simulink model "itki"  (R2019b)
settings: Solver=VariableStepAuto  StartTime=0.0  StopTime=1000  RelTol=1e-3
model workspace (MAT data in the model file):
  itki = [0 1000 1800 2300 2400 2350 2400 2600 2300 2250 2200 750 150 100 20]
undefined symbols (not defined in the file): Earth, magnitude, WGS84
libraries: dspsrcs4 x3, aerolibfltsims x2, simulink x1, sharedtransform x1, aerolibtransform2 x1
settings Model: Creator=LENOVO  LastModifiedBy=LENOVO

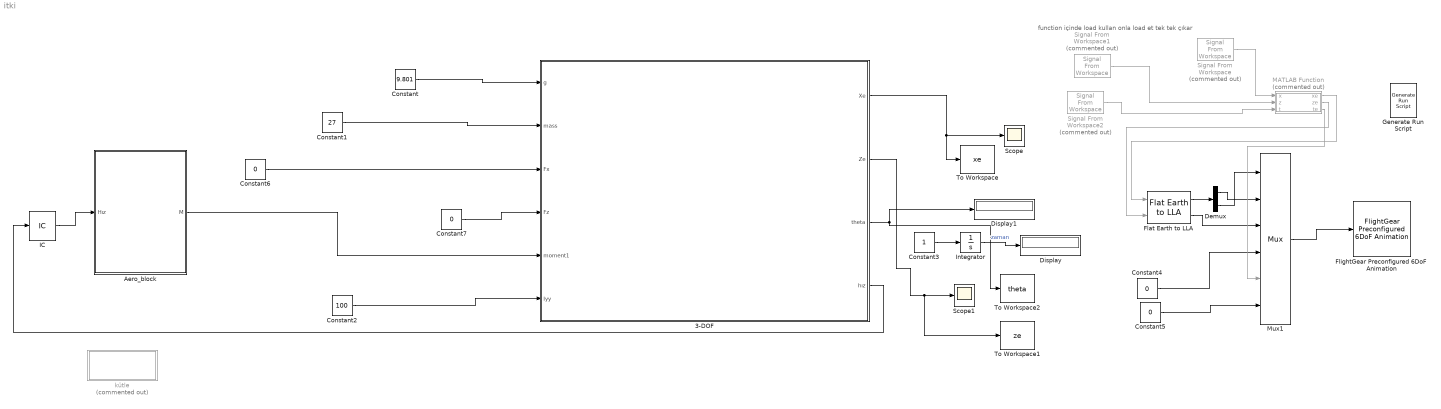
== system itki ==
  note: function içinde load kullan onla load et tek tek çıkar
  3-DOF : Subsystem
  Aero_block : Subsystem
  Constant : Constant  Value=9.801
  Constant1 : Constant  Value=27
  Constant2 : Constant  Value=100
  Constant3 : Constant
  Constant{4..7} (4 alike) : Constant  Value=0
  Demux : Demux  Outputs=2
  Display : Display
  Display1 : Display
  Flat Earth to LLA : aerolibtransform2/Flat Earth to LLA  units=Metric (MKS)  ptype=Earth (WGS84)  F=1/298.257223563  R=6378137  LL0=[0 10]  psi=0
  FlightGear Preconfigured 6DoF Animation : aerolibfltsims/FlightGear Preconfigured 6DoF Animation  xFlightGearVersion=v2018.3  DestinationIpAddress=127.0.0.1  DestinationPort=5502  SampleTime=1/30  packetVersion=24
      settings: SourceProductName=Aerospace Blockset
  Generate Run Script : aerolibfltsims/Generate Run Script  Architecture=Win64  dataFlow=Send  GeometryModelName=HL20  AirportId=KSFO  RunwayId=10L  InitialAltitude=7224  InitialHeading=113  OffsetDistance=4.72  OffsetAzimuth=0  InstallScenery=off  DisableShaders=on  OriginAddress=127.0.0.1  DestinationPort=5502  OriginPort=5505  LocalAddress=127.0.0.1  OutputFileName=runfg.bat  FlightGearBaseDirectory=C:\Program Files\FlightGear 2020.3
  IC : InitialCondition  Value=100
  Integrator : Integrator
  MATLAB Function : MATLAB Function  Commented=on  TreatAsAtomicUnit=on
  Mux1 : Mux  Inputs=6
  Scope : Scope
  Scope1 : Scope
  Signal From Workspace : dspsrcs4/Signal From Workspace  Commented=on  X=out.xe  Ts=0.1  nsamps=1  OutputAfterFinalValue=Setting to zero  ignoreOrWarnInputAndFrameLengths=off  OutputFrames=off
  Signal From Workspace1 : dspsrcs4/Signal From Workspace  Commented=on  X=out.ze  Ts=0.1  nsamps=1  OutputAfterFinalValue=Setting to zero  ignoreOrWarnInputAndFrameLengths=off  OutputFrames=off
  Signal From Workspace2 : dspsrcs4/Signal From Workspace  Commented=on  X=out.theta  Ts=0.1  nsamps=1  OutputAfterFinalValue=Setting to zero  ignoreOrWarnInputAndFrameLengths=off  OutputFrames=off
  To Workspace : ToWorkspace  VariableName=xe  SampleTime=0.1
      settings: Save2DSignal=2-D array (concatenate along first dimension)
  To Workspace1 : ToWorkspace  VariableName=ze  SampleTime=0.1
      settings: Save2DSignal=2-D array (concatenate along first dimension)
  To Workspace2 : ToWorkspace  VariableName=theta  SampleTime=0.1
      settings: Save2DSignal=2-D array (concatenate along first dimension)
  kütle : Subsystem  Commented=on
  wires:
  Constant/1 -> 3-DOF/1(g)
  Constant1/1 -> 3-DOF/2(mass)
  Constant6/1 -> 3-DOF/3(Fx)
  Aero_block/1(M) -> 3-DOF/5(moment1)
  Constant2/1 -> 3-DOF/6(Iyy)
  3-DOF/2(Ze) -> To Workspace1/1, Scope1/1
  Constant3/1 -> Integrator/1
  Integrator/1 -> Display/1  "zaman"
  Flat Earth to LLA/1 -> Demux/1
  Demux/1 -> Mux1/2
  Demux/2 -> Mux1/1
  Flat Earth to LLA/2 -> Mux1/3
  Mux1/1 -> FlightGear Preconfigured 6DoF Animation/1
  Constant5/1 -> Mux1/6
  Signal From Workspace1/1 -> MATLAB Function/2(z)
  Signal From Workspace/1 -> MATLAB Function/1(x)
  Signal From Workspace2/1 -> MATLAB Function/3(t)
  Constant4/1 -> Mux1/4
  3-DOF/1(Xe) -> To Workspace/1, Scope/1
  3-DOF/3(theta) -> Display1/1, To Workspace2/1
  MATLAB Function/1(xe) -> Flat Earth to LLA/1
  MATLAB Function/2(ze) -> Flat Earth to LLA/2
  MATLAB Function/3(te) -> Mux1/5
  Constant7/1 -> 3-DOF/4(Fz)
  3-DOF/4(hız) -> IC/1
  IC/1 -> Aero_block/1(Hız)

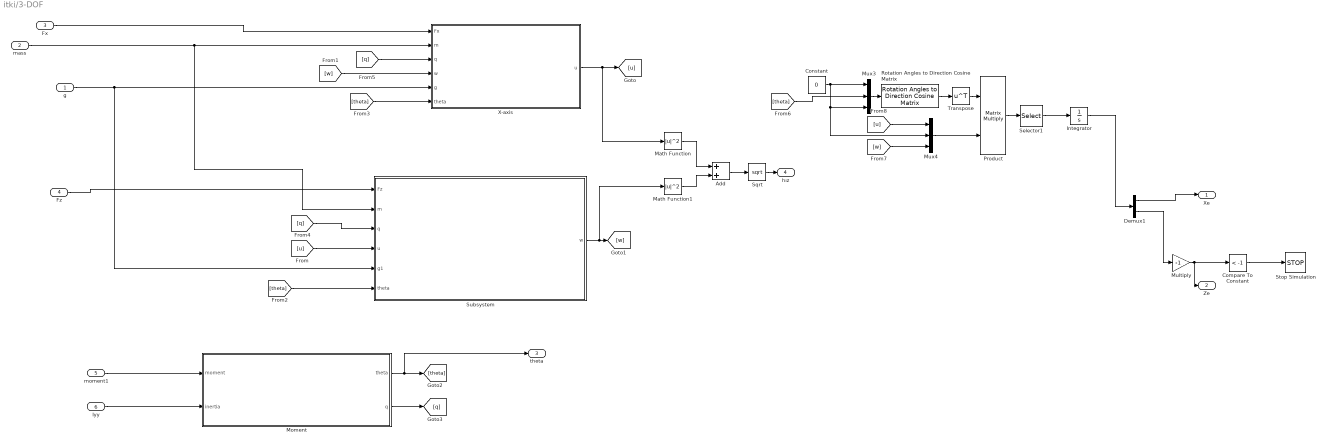
== system itki/3-DOF ==
  g : Inport
  mass : Inport  Port=2
  Fx : Inport  Port=3
  Fz : Inport  Port=4
  moment1 : Inport  Port=5
  Iyy : Inport  Port=6
  Add : Sum
  Compare To Constant : simulink/Logic and Bit Operations/Compare To Constant  relop=<  const=-1  OutDataTypeStr=boolean
  Constant : Constant  Value=0
  Demux1 : Demux  Outputs=2
  Integrator : Integrator
  Math Function : Math  Operator=magnitude^2  SignedPower=off  SaturateOnIntegerOverflow=on
  Math Function1 : Math  Operator=magnitude^2  SignedPower=off  SaturateOnIntegerOverflow=on
  Moment : Subsystem
  Multiply : Gain  Gain=-1
  Mux3 : Mux  Inputs=3
  Mux4 : Mux  Inputs=3
  Product : Product  Multiplication=Matrix(*)  SaturateOnIntegerOverflow=on  OutDataTypeStr=Inherit: Same as first input
  Rotation Angles to Direction Cosine Matrix : sharedtransform/Rotation Angles to Direction Cosine Matrix  rotationOrder=ZYX  aMode=aMode
      settings: SourceProductBaseCode=AE
  Selector1 : Selector  InputPortWidth=3  IndexOptions=Index vector (dialog)  Indices=[1 3]  OutputSizes=1
  Sqrt : Sqrt  SaturateOnIntegerOverflow=on
  Stop Simulation : Stop
  Subsystem : Subsystem
  Transpose : Math  Operator=transpose  SaturateOnIntegerOverflow=on
  X-axis : Subsystem
  Xe : Outport
  Ze : Outport  Port=2
  theta : Outport  Port=3
  hız : Outport  Port=4
  wires:
  moment1/1 -> Moment/1(moment)
  [u] -> Subsystem/4(u)
  [theta] -> X-axis/6(theta)
  mass/1 -> Subsystem/2(m), X-axis/2(m)
  g/1 -> Subsystem/5(g1), X-axis/5(g)
  [theta] -> Subsystem/6(theta)
  Subsystem/1(w) -> Math Function1/1, [w]
  Fz/1 -> Subsystem/1(Fz)
  Fx/1 -> X-axis/1(Fx)
  [w] -> X-axis/4(w)
  X-axis/1(u) -> Math Function/1, [u]
  Iyy/1 -> Moment/2(inertia)
  Moment/2(q) -> [q]
  [q] -> Subsystem/3(q)
  [q] -> X-axis/3(q)
  Math Function/1 -> Add/1
  Math Function1/1 -> Add/2
  Add/1 -> Sqrt/1
  Mux4/1 -> Product/2
  Rotation Angles to Direction Cosine Matrix/1 -> Transpose/1
  Product/1 -> Selector1/1
  [w] -> Mux4/3
  [u] -> Mux4/1
  Selector1/1 -> Integrator/1
  Mux3/1 -> Rotation Angles to Direction Cosine Matrix/1
  [theta] -> Mux3/2
  Transpose/1 -> Product/1
  Constant/1 -> Mux3/1, Mux4/2, Mux3/3
  Integrator/1 -> Demux1/1
  Demux1/1 -> Xe/1
  Demux1/2 -> Multiply/1
  Multiply/1 -> Compare To Constant/1, Ze/1
  Compare To Constant/1 -> Stop Simulation/1
  Moment/1(theta) -> theta/1, [theta]
  Sqrt/1 -> hız/1

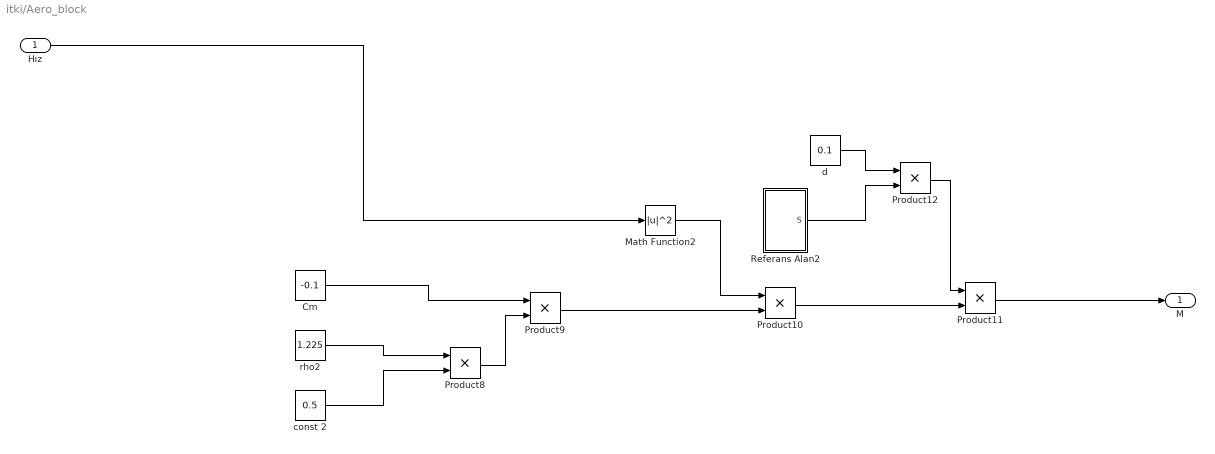
== system itki/Aero_block ==
  Hız : Inport
  Cm : Constant  Value=-0.1
  Math Function2 : Math  Operator=magnitude^2  SignedPower=off  SaturateOnIntegerOverflow=on
  Product{8..12} (5 alike) : Product
  Referans Alan2 : Subsystem
  const 2 : Constant  Value=0.5
  d : Constant  Value=0.1
  rho2 : Constant  Value=1.225
  M : Outport
  wires:
  const 2/1 -> Product8/2
  rho2/1 -> Product8/1
  Cm/1 -> Product9/1
  Product8/1 -> Product9/2
  Hız/1 -> Math Function2/1
  Product9/1 -> Product10/2
  Math Function2/1 -> Product10/1
  Product10/1 -> Product11/2
  Product11/1 -> M/1
  d/1 -> Product12/1
  Referans Alan2/1(S) -> Product12/2
  Product12/1 -> Product11/1

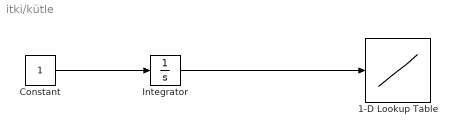
== system itki/kütle ==
  1-D Lookup Table : Lookup_n-D  NumberOfTableDimensions=1  BreakpointsForDimension1=[0 3]  Table=[10.5 6.531]  InternalRulePriority=Speed  RndMeth=Simplest  InputSameDT=on
  Constant : Constant
  Integrator : Integrator
  wires:
  Constant/1 -> Integrator/1
  Integrator/1 -> 1-D Lookup Table/1

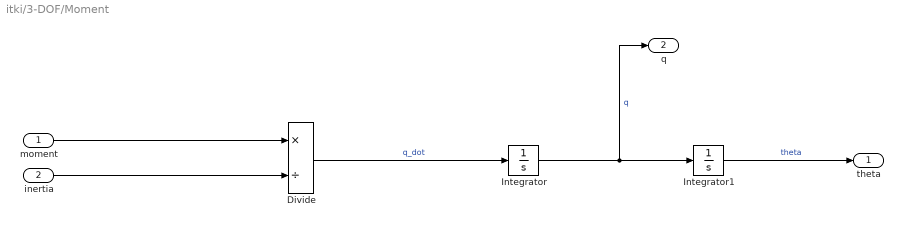
== system itki/3-DOF/Moment ==
  moment : Inport
  inertia : Inport  Port=2
  Divide : Product  Inputs=*/
  Integrator : Integrator
  Integrator1 : Integrator  InitialCondition=70*pi/180
  theta : Outport
  q : Outport  Port=2
  wires:
  Integrator/1 -> q/1, Integrator1/1  "q"
  moment/1 -> Divide/1
  Divide/1 -> Integrator/1  "q_dot"
  Integrator1/1 -> theta/1  "theta"
  inertia/1 -> Divide/2

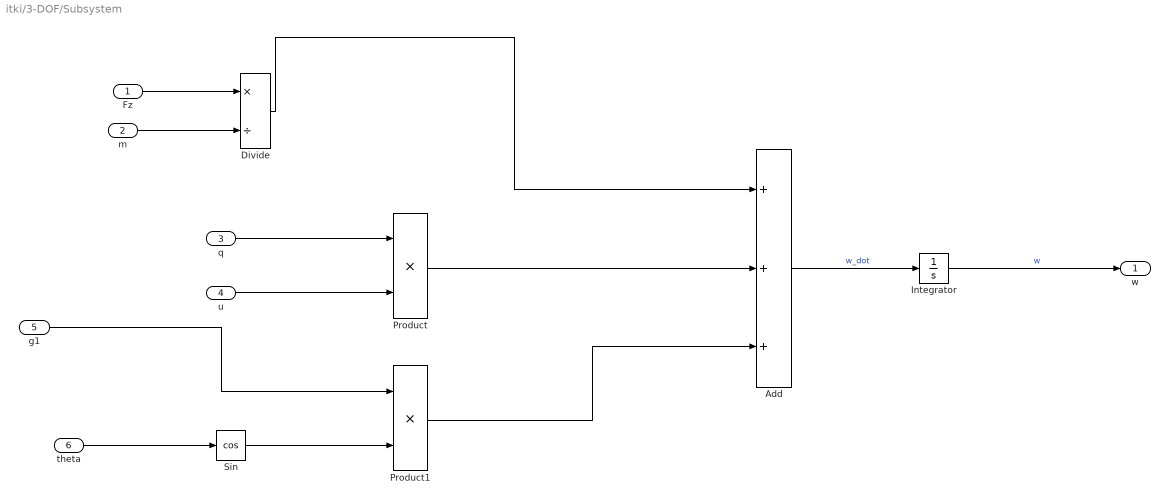
== system itki/3-DOF/Subsystem ==
  Fz : Inport
  m : Inport  Port=2
  q : Inport  Port=3
  u : Inport  Port=4
  g1 : Inport  Port=5
  theta : Inport  Port=6
  Add : Sum  Inputs=+++
  Divide : Product  Inputs=*/
  Integrator : Integrator
  Product : Product
  Product1 : Product
  Sin : Trigonometry  Operator=cos
  w : Outport
  wires:
  theta/1 -> Sin/1
  Divide/1 -> Add/1
  Add/1 -> Integrator/1  "w_dot"
  Product1/1 -> Add/3
  Product/1 -> Add/2
  q/1 -> Product/1
  u/1 -> Product/2
  Sin/1 -> Product1/2
  g1/1 -> Product1/1
  m/1 -> Divide/2
  Integrator/1 -> w/1  "w"
  Fz/1 -> Divide/1

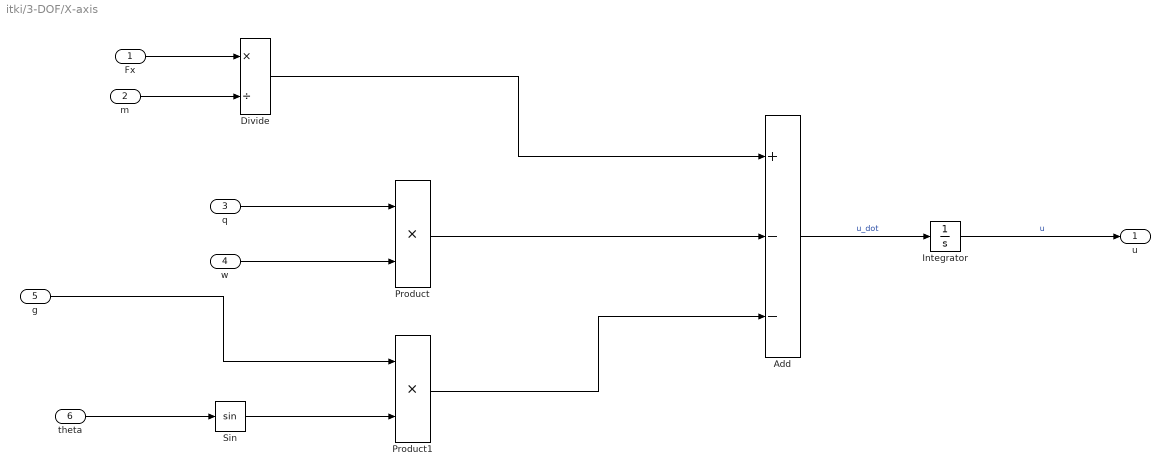
== system itki/3-DOF/X-axis ==
  Fx : Inport
  m : Inport  Port=2
  q : Inport  Port=3
  w : Inport  Port=4
  g : Inport  Port=5
  theta : Inport  Port=6
  Add : Sum  Inputs=+--
  Divide : Product  Inputs=*/
  Integrator : Integrator
  Product : Product
  Product1 : Product
  Sin : Trigonometry
  u : Outport
  wires:
  q/1 -> Product/1
  Product/1 -> Add/2
  Sin/1 -> Product1/2
  m/1 -> Divide/2
  Add/1 -> Integrator/1  "u_dot"
  w/1 -> Product/2
  Fx/1 -> Divide/1
  Integrator/1 -> u/1  "u"
  Product1/1 -> Add/3
  Divide/1 -> Add/1
  g/1 -> Product1/1
  theta/1 -> Sin/1

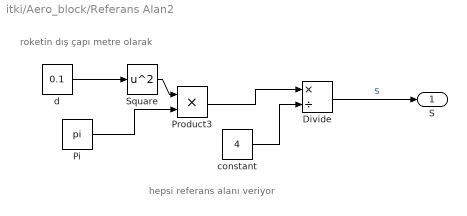
== system itki/Aero_block/Referans Alan2 ==
  note: roketin dış çapı metre olarak
  note: hepsi referans alanı veriyor
  Divide : Product  Inputs=*/
  Pi : Constant  Value=pi  OutDataTypeStr=Inherit: Inherit via back propagation
  Product3 : Product
  Square : Math  Operator=square  SignedPower=off  SaturateOnIntegerOverflow=on
  "constant " : Constant  Value=4
  d : Constant  Value=0.1
  S : Outport
  wires:
  Pi/1 -> Product3/2
  "constant "/1 -> Divide/2
  Product3/1 -> Divide/1
  Divide/1 -> S/1  "S"
  Square/1 -> Product3/1
  d/1 -> Square/1

== matlab function itki/MATLAB Function ==
  data: x input; xe output; z input; t input; ze output; te output
function [xe,ze,te] = fcn(x,z,t)
xe=[x(1,1) ;x(1,1) ; x(1,1)];
ze=-z(1,1);
te=t(1,1);
end
